simulink model "Inc_Counter"  (R2021a)
settings: Solver=VariableStepAuto  StartTime=0.0  StopTime=10.0  RelTol=1e-3
settings Model: Creator=Moamen_Hamed  LastModifiedBy=Moamen_Hamed

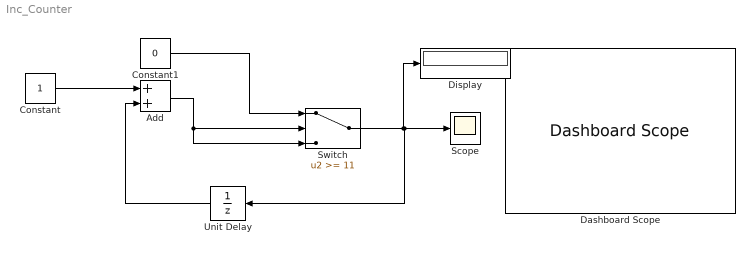
== system Inc_Counter ==
  Add : Sum
  Constant : Constant
  Constant1 : Constant  Value=0
  Dashboard Scope : DashboardScope
  Display : Display
  Scope : Scope
  Switch : Switch  Threshold=11
  Unit Delay : UnitDelay  SampleTime=-1  HasFrameUpgradeWarning=on
  wires:
  Constant/1 -> Add/1
  Unit Delay/1 -> Add/2
  Switch/1 -> Display/1, Scope/1, Unit Delay/1
  Add/1 -> Switch/3, Switch/2
  Constant1/1 -> Switch/1
